simulink model "MotionLab_DigitalTwin"  (R2024b)
settings: Solver=ode3  StartTime=0.0  StopTime=inf  FixedStep=Ts  RelTol=1e-3  AbsTol=1e-3
model workspace: external: MATLAB File .\Parameters.m (data not in the file)
values from neighbouring files (symbols this model uses):
  L2 = 830e-3    (= 0.83)    [Robot_parameters.m]
  L3 = 1160e-3    (= 1.16)    [Robot_parameters.m]
  L4 = 250e-3    (= 0.25)    [Robot_parameters.m]
undefined symbols (not defined in the file or in its folder): smiData, smiDataBig, smiDataBigTop, smiDataRobot, Var, X, Y, Z
libraries: sm_lib x490, nesl_utility x87, slrealtimeutilitieslib x1, slrealtimeiplib x1, aerolibanimutils x1
(part 15 of 15)

== matlab function MotionLab_DigitalTwin/VHT eMotion-8000 Stewart Platform/Motion Control System/MotionGen ==
  data: surge input; motion output; R_top output; p_top output; sway input; heave input; roll input; pitch input; yaw input
function [motion, R_top, p_top] = platform_motion(surge, sway, heave, roll, pitch, yaw)
    % platform_motion_udp - Generate platform motion data using UDP feedback
    %
    % Input:
    %   udpData - A structure containing the UDP feedback variables with fields:
    %             em8000_surge, em8000_sway, em8000_heave, 
    %             em8000_roll, em8000_pitch, em8000_yaw, 
    %             (and optionally velocities and accelerations if needed)
    %
    % Outputs:
    %   motion - A 6x1 vector [surge; sway; heave; roll; pitch; yaw]
    %   p_top  - A 3x1 vector representing the translational position [x; y; z]
    %   R_top  - A 3x3 rotation matrix computed from the Euler angles
    %
    % Example usage:
    %   udpData = getUDPData(); % Assume this function reads from UDP
    %   [motion, R_top, p_top] = platform_motion_udp(udpData);
    
    % Extract translational positions [m]
    x = -surge;
    y = -sway;
    z = -heave;
    
    % Extract Euler angles [rad]
    %roll  = roll;
    %pitch = pitch;
    %yaw   = yaw;
    
    % Form the motion vector: translations and rotations
    motion = [x; y; z; roll; pitch; yaw];
    
    % Define the top position vector (only translations)
    p_top = [x; y; z];
    
    % Compute the rotation matrix.
    % Assuming the eul2rotm function expects angles in the order [yaw, pitch, roll]
    R_top = eul2rotm([yaw, pitch, roll]);
end
